simulink model "DC_motor_Ex_1"  (R2025a)
settings: Solver=VariableStepAuto  StartTime=0.0  StopTime=70.0  RelTol=1e-3
undefined symbols (not defined in the file or in its folder): K_I_gain, K_P, Load
settings Model: Creator=dimpa  LastModifiedBy=Mads2
settings DebuggingCC: UnconnectedInputMsg=warning  UnconnectedOutputMsg=warning  UnconnectedLineMsg=warning
settings ModelReferenceCC: EnableRefExpFcnMdlSchedulingChecks=on
settings RTWCC: GPUComputeCapability=3.5  DLArmComputeVersion=19.05

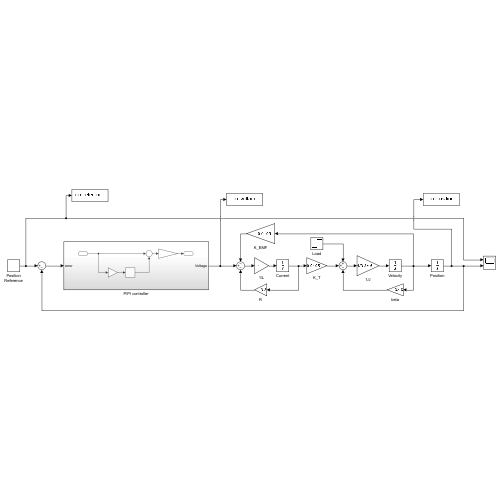
[thumbnail: Simulink's stored preview of the top-level diagram]
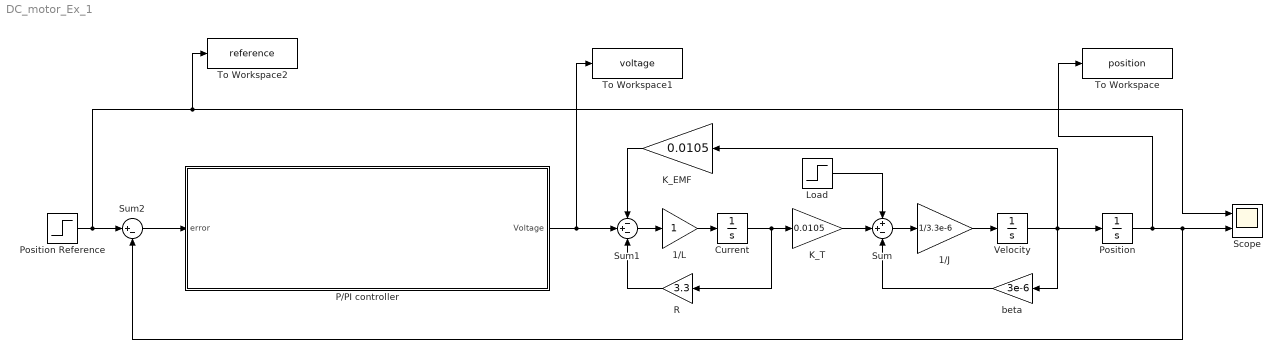
== system DC_motor_Ex_1 ==
  1/J : Gain  Gain=1/3.3e-6
  1/L : Gain
  Current : Integrator
  K_EMF : Gain  Gain=0.0105
  K_T : Gain  Gain=0.0105
  Load : Step  Time=10  After=Load  SampleTime=0
  P/PI controller : Subsystem
  Position : Integrator
  Position Reference : Step  SampleTime=0.001
  R : Gain  Gain=3.3
  Scope : Scope  NumInputPorts=2
      settings: ActiveDisplayYMinimum=-0.26914132956200432  ActiveDisplayYMaximum=1.1915581776731075
  Sum : Sum  Inputs=++-
  Sum1 : Sum  Inputs=-+-
  Sum2 : Sum  Inputs=|+-
  To Workspace : ToWorkspace  VariableName=position  SaveFormat=Timeseries  SampleTime=-1
  To Workspace1 : ToWorkspace  VariableName=voltage  SaveFormat=Timeseries  SampleTime=-1
  To Workspace2 : ToWorkspace  VariableName=reference  SaveFormat=Timeseries  SampleTime=-1
  Velocity : Integrator
  beta : Gain  Gain=3e-6
  wires:
  Velocity/1 -> K_EMF/1, beta/1, Position/1
  beta/1 -> Sum/3
  Sum/1 -> 1/J/1
  K_T/1 -> Sum/2
  Current/1 -> K_T/1, R/1
  K_EMF/1 -> Sum1/1
  R/1 -> Sum1/3
  Sum1/1 -> 1/L/1
  1/J/1 -> Velocity/1
  P/PI controller/1(Voltage) -> To Workspace1/1, Sum1/2
  Position Reference/1 -> To Workspace2/1, Scope/1, Sum2/1
  Position/1 -> To Workspace/1, Scope/2, Sum2/2
  Sum2/1 -> P/PI controller/1(error)
  Load/1 -> Sum/1
  1/L/1 -> Current/1

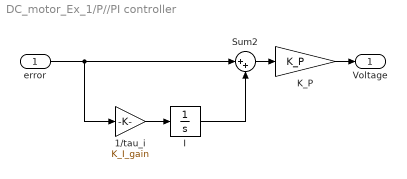
== system DC_motor_Ex_1/P//PI controller ==
  error : Inport
  1/tau_i : Gain  Gain=K_I_gain
  I : Integrator
  K_P : Gain  Gain=K_P
  Sum2 : Sum  Inputs=|++
  Voltage : Outport
  wires:
  error/1 -> 1/tau_i/1, Sum2/1
  Sum2/1 -> K_P/1
  1/tau_i/1 -> I/1
  I/1 -> Sum2/2
  K_P/1 -> Voltage/1
